simulink model "P2D_Overall"  (R2022a)
settings: Solver=VariableStepAuto  StartTime=0.0  StopTime=1  RelTol=1e-3
model workspace (MAT data in the model file):
  AN.EqPotentialHandle = 'E_eqGraphite'
  AN.i_oHandle = 'i_oC6'
  AN.sigmaHandle = 'sigmaC6'
  AN.D_oHandle = 'D_o_Graphite'
  AN.k_o = 3.80589129595e-09
  AN.alpha_a = 0.5
  AN.alpha_c = 0.5
  AN.C_dl = 3e-06
  AN.R_SEI = 0.00733702042142
  AN.sigma = 100
  AN.D_o = 3e-13
  AN.MW = 72.0642
  AN.MW_Lith = 79.0052
  AN.specCap = 350
  AN.rho = 2266
  AN.c_p = 720
  AN.k = 0.6
  AN.C_Li_max = 28.4851292094
  AN.del_z = 0.316227766017
  AN.del_y = 0.316227766017
  AN.L = 0.0001
  AN.r_p = 1.25e-05
  AN.eps_ed = 0.320700992698
  AN.eps_b = 0.172
  AN.A_geo = 1
  AN.gamma_brug = 1
  AN.alpha_brug = 1.5
  AN.del_x = 1e-05
  AN.x_vec = [5e-06 1.5e-05 2.5e-05 3.5e-05 4.5e-05 5.5e-05 6.5e-05 7.5e-05 8.5e-05 9.5e-05]
  AN.x_half_vec = [0 1e-05 2e-05 3e-05 4e-05 5e-05 6e-05 7e-05 8e-05 9e-05 0.0001]
  AN.del_r = 1.25e-06
  AN.r_vec = [6.25e-07 1.875e-06 3.125e-06 4.375e-06 5.625e-06 6.875e-06 8.125e-06 9.375e-06 1.0625e-05 1.1875e-05]
  AN.r_half_vec = [0 1.25e-06 2.5e-06 3.75e-06 5e-06 6.25e-06 7.5e-06 8.75e-06 1e-05 1.125e-05 1.25e-05]
  AN.eps_el = 0.507299007302
  AN.A_c = 0.1
  AN.Vol = 1e-05
  AN.dVol = 1e-06
  AN.V_sphere = 8.18123086872e-15
  AN.V_ed = 3.20700992698e-06
  AN.V_el = 5.07299007302e-06
  AN.dVol_el = 5.07299007302e-07
  AN.Np_tot = 391996018.501
  AN.Np_CV = 39199601.8501
  AN.A_surf = 1.96349540849e-09
  AN.A_surf_tot = 0.769682382475
  AN.A_surf_CV = 0.0769682382475
  AN.A_s = 76968.2382475
  AN.dVol_r = [8.18123086872e-18; 5.72686160811e-17; 1.55443386506e-16; 3.02705542143e-16; 4.99055082992e-16; 7.44492009054e-16; 1.03901632033e-15; 1.38262801681e-15; 1.77532709851e-15; 2.21711356542e-15]
  AN.Cap = 2.44837153197
  A_ROM = [0.499929926021  0.500277672565  -0.0239600367005  -0.00259805630083  0.0203144018753  -0.00104534668098  0.00239552572438  -0.000195556886825  -0.000910447986479  -7.26333553818e-05; -0.499881297031  -0.499911034591  -0.0239719306113  -0.00260057015341  0.0203228961157  -0.00104589940542  0.00239669880443  -0.000195607988547  -0.000910809830954  -7.2671508135e-05; 0.0251047076349  -0.0250959457318  0.987171638248  -0.00653392621931  0.0197762134396  -0.00226585752594  0.00331411596577  -0.000147058370919  -0.00053836838787  -4.66457939345e-05; -0.00955893642669  0.00955505732616  0.0123516491588  1.00099526202  -0.000703718615196  -0.000890966549299  0.00221912313357  -0.000101956509457  7.04769385898e-06  -4.36093200247e-06; 0.0212890549632  -0.0212815772566  -0.0230812878959  0.0308592552326  0.873793995824  -0.00311715755808  -0.0172138406461  0.00328787148246  0.0140204587776  0.001112904288; 0.00443110495424  -0.0044294863981  -0.0044884586816  0.00438260533447  -0.0577192270273  0.812800487273  0.104548665471  0.0343410474239  0.0440871519918  0.00415412252809; -0.00321407179364  0.00321296141751  0.00318368985247  -0.00520269619945  0.040746062799  0.244510956525  0.815824906709  -0.0403403883233  -0.00463968834278  0.000324235347067; 0.000411908248218  -0.000411728572718  -0.000450970628534  -0.000520935242046  -0.00616085036225  -0.0459578894952  0.0901889133124  0.991986422474  -0.0379589014963  -0.00193613802868; -0.000841734726446  0.000841438210464  0.000843091769749  -0.00117615267803  0.0106356056607  0.0898474768325  -0.118952953028  0.086084355624  0.424203198737  -0.0291971042377; -7.03725269776e-05  7.03386483629e-05  8.0548900339e-05  0.000189879859473  0.00113672762497  0.00528200920844  -0.0130569138272  -0.00245106078529  -0.137785624495  0.985398155877]
  A_est = [0.499929926021  0.500277672565  -0.0239600367005  -0.00259805630083  0.0203144018753  -0.00104534668098  0.00239552572438  -0.000195556886825  -0.000910447986479  -7.26333553818e-05; -0.499881297031  -0.499911034591  -0.0239719306113  -0.00260057015341  0.0203228961157  -0.00104589940542  0.00239669880443  -0.000195607988547  -0.000910809830954  -7.2671508135e-05; 0.0251047076349  -0.0250959457318  0.987171638248  -0.00653392621931  0.0197762134396  -0.00226585752594  0.00331411596577  -0.000147058370919  -0.00053836838787  -4.66457939345e-05; -0.00955893642669  0.00955505732616  0.0123516491588  1.00099526202  -0.000703718615196  -0.000890966549299  0.00221912313357  -0.000101956509457  7.04769385898e-06  -4.36093200247e-06; 0.0212890549632  -0.0212815772566  -0.0230812878959  0.0308592552326  0.873793995824  -0.00311715755808  -0.0172138406461  0.00328787148246  0.0140204587776  0.001112904288; 0.00443110495424  -0.0044294863981  -0.0044884586816  0.00438260533447  -0.0577192270273  0.812800487273  0.104548665471  0.0343410474239  0.0440871519918  0.00415412252809; -0.00321407179364  0.00321296141751  0.00318368985247  -0.00520269619945  0.040746062799  0.244510956525  0.815824906709  -0.0403403883233  -0.00463968834278  0.000324235347067; 0.000411908248218  -0.000411728572718  -0.000450970628534  -0.000520935242046  -0.00616085036225  -0.0459578894952  0.0901889133124  0.991986422474  -0.0379589014963  -0.00193613802868; -0.000841734726446  0.000841438210464  0.000843091769749  -0.00117615267803  0.0106356056607  0.0898474768325  -0.118952953028  0.086084355624  0.424203198737  -0.0291971042377; -7.03725269776e-05  7.03386483629e-05  8.0548900339e-05  0.000189879859473  0.00113672762497  0.00528200920844  -0.0130569138272  -0.00245106078529  -0.137785624495  0.985398155877]
  B_ROM = [0.250272154511; 0.25037068325; 0.000587633015339; 2.64174643029e-05; -4.66234471071e-05; 1.60139296354e-07; -1.87943663585e-07; -2.31065441941e-09; 7.21267341548e-09; 1.30921415116e-10]
  B_est = [0.250272154511; 0.25037068325; 0.000587633015339; 2.64174643029e-05; -4.66234471071e-05; 1.60139296354e-07; -1.87943663585e-07; -2.31065441941e-09; 7.21267341548e-09; 1.30921415116e-10]
  CA.EqPotentialHandle = 'E_eqNMC'
  CA.i_oHandle = 'i_oC6'
  CA.sigmaHandle = 'sigmaNMC'
  CA.D_oHandle = 'D_o_NMC532'
  CA.k_o = 9.72997022034e-10
  CA.alpha_a = 0.5
  CA.alpha_c = 0.5
  CA.C_dl = 1e-06
  CA.R_SEI = 0.00611911635272
  CA.sigma = 3.8
  CA.D_o = 5e-13
  CA.MW = 89.61275
  CA.MW_Lith = 96.55375
  CA.specCap = 170
  CA.rho = 2739.6961
  CA.c_p = 720
  CA.k = 0.6
  CA.C_Li_max = 40.5441490868
  CA.del_z = 0.316227766017
  CA.del_y = 0.316227766017
  CA.L = 0.0001
  CA.r_p = 5e-06
  CA.eps_ed = 0.442994582877
  CA.eps_b = 0.259
  CA.A_geo = 1
  CA.gamma_brug = 1
  CA.alpha_brug = 1.5
  CA.del_x = 1e-05
  CA.x_vec = [0.000135 0.000145 0.000155 0.000165 0.000175 0.000185 0.000195 0.000205 0.000215 0.000225]
  CA.x_half_vec = [0.00013 0.00014 0.00015 0.00016 0.00017 0.00018 0.00019 0.0002 0.00021 0.00022 0.00023]
  CA.del_r = 5e-07
  CA.r_vec = [2.5e-07 7.5e-07 1.25e-06 1.75e-06 2.25e-06 2.75e-06 3.25e-06 3.75e-06 4.25e-06 4.75e-06]
  CA.r_half_vec = [0 5e-07 1e-06 1.5e-06 2e-06 2.5e-06 3e-06 3.5e-06 4e-06 4.5e-06 5e-06]
  CA.eps_el = 0.298005417123
  CA.A_c = 0.1
  CA.Vol = 1e-05
  CA.dVol = 1e-06
  CA.V_sphere = 5.23598775598e-16
  CA.V_ed = 4.42994582877e-06
  CA.V_el = 2.98005417123e-06
  CA.dVol_el = 2.98005417123e-07
  CA.Np_tot = 8460573315.33
  CA.Np_CV = 846057331.533
  CA.A_surf = 3.14159265359e-10
  CA.A_surf_tot = 2.65796749726
  CA.A_surf_CV = 0.265796749726
  CA.A_s = 265796.749726
  CA.dVol_r = [5.23598775598e-19; 3.66519142919e-18; 9.94837673637e-18; 1.93731546971e-17; 3.19395253115e-17; 4.76474885794e-17; 6.6497044501e-17; 8.84881930761e-17; 1.13620934305e-16; 1.41895268187e-16]
  CA.Cap = 4.81377102891
  CONS.F = 96485338.3
  CONS.R = 8314.472
  CONS.T = 298.15
  C_ROM = [-0.00545632264226 0.00546070995292 -0.00275985407975 -0.0016343921732 -0.000623828440853 -0.00060095083733 0.000490320954801 1.36778683108e-05 0.000375099015739 1.69573705691e-05]
  C_est = [-0.00545632264226 0.00546070995292 -0.00275985407975 -0.0016343921732 -0.000623828440853 -0.00060095083733 0.000490320954801 1.36778683108e-05 0.000375099015739 1.69573705691e-05]
  C_plant = [0 0 -1 0 0 0 0 0 0 0 0 0 0 0 0 0 0 0 0 0 0 0 0 0 0 0 0 0 0 0 0 0 0 0 0 0 0 0 0 0 0 0 0 0 0 0 0 0 0 0 0 0 0 0 0 0 0 0 0 0 0 0 0 0 0 0 0 0 0 0 0 0 0 0 0 0 0 0 0 0 0 0 0 0 0 0 0 0 0 0 0 0 0 0 0 0 0 0 0 0 0 0 0 0 0 0 0 0 0 0 0 0 0 0 0 0 0 0 0 0 0 0 0 0 0 0 0 0 0 0 0 0 0 0 0 0 0 0 0 0 0 0 0 0 0 0 0 0 0 0 0 0 0 0 0 0 0 0 0 0 0 0 0 0 0 0 0 0 0 0 0 0 0 0 0 0 0 0 0 0 0 0 0 0 0 0 0 0 0 0 0 0 0 0 0 0 0 0 0 0 0 0 0 0 0 0 0 0 0 0 0 0 0 0 0 0 0 0 0 0 0 0 0 0 0 0 0 0 0 0 0 0 0 0 0 0 0 0 0 0 0 0 0 0 0 0 0 0 0 0 0 0 0 0 0 0 0 0 0 0 0 0 0 0 0 0 0 0 0 0 0 0 0 0 0 0 0 0 0 0 0 0 0 0 0 0 0 0 0 0 0 0 0 0 0 0 0 0 0 0 0 0 0 0 0 0 0 0 0 0 0 0 0 0 0 0 0 0 0 0 0 0 0 0 0 0 0 0 0 0 0 0 0 0 0 0 0 0 0 0 1 0 0 0 0 0 0 0 0 0 0 0 0 0 0]
  EL.tf_numHandle = 'transferenceNumber'
  EL.ActivityHandle = 'activity'
  EL.D_o_Li_ionHandle = 'D_oLiion'
  EL.kappaHandle = 'kappa'
  EL.D_o_Li_ion = 7.5e-11
  EL.kappa = 0.28
  EL.C = 1
  EL.tf_num = 0.363
  EL.Activity = 1
  EL.rho = 2266
  EL.c_p = 720
  EL.k = 470
  EL.gamma_brug = 1
  EL.alpha_brug = 1.5
  FLAG.AN_LI_FOIL = 0
  FLAG.CA_LI_FOIL = 0
  FLAG.R_AN = 1
  FLAG.R_CA = 1
  FLAG.COE = 0
  FLAG.T_BC_AN = 4
  FLAG.T_BC_CA = 4
  FLAG.CV_CONV = 0
  FLAG.HEAT_GEN_TOTAL = 1
  FLAG.HEAT_GEN_IONIC = 1
  FLAG.HEAT_GEN_ELECTRIC = 1
  FLAG.HEAT_GEN_RXN = 1
  FLAG.HEAT_GEN_CHEM_RXN = 0
  FLAG.V_SEI = 1
  FLAG.SEI_growth = 0
  FLAG.HeatGen = 0
  FLAG.Bruggeman = 0
  FLAG.BRUG_ED = 1
  FLAG.BRUG_EL = 1
  FLAG.BRUG_sigma = 1
  FLAG.BRUG_kappa = 1
  FLAG.BRUG_activity = 0
  FLAG.BRUG_D_Liion = 1
  FLAG.BRUG_tf_num = 0
  FLAG.BRUG_D_o_AN = 0
  FLAG.BRUG_D_o_CA = 0
  FLAG.Newman_i_o = 1
  FLAG.preDefined_C_max = 1
  FLAG.CONSTANT_PROPS_FROM_HANDLES = 0
  FLAG.VARIABLE_PROPS_FROM_HANDLES = 0
  FLAG.VARIABLE_kappa = 1
  FLAG.VARIABLE_activity = 0
  FLAG.VARIABLE_D_Liion = 0
  FLAG.VARIABLE_tf_num = 0
  FLAG.VARIABLE_D_o_AN = 0
  FLAG.VARIABLE_D_o_CA = 0
  FLAG.SaveSolnDiscreteTime = 1
  FLAG.SaveSystemForEst = 0
  FLAG.doPostProcessing = 1
  FLAG.ReduceSolnTime = 0
  FLAG.Plot = 0
  FLAG.PRBS_predefinded = 0
  Iden = [1  0  0  0  0  0  0  0  0  0; 0  1  0  0  0  0  0  0  0  0; 0  0  1  0  0  0  0  0  0  0; 0  0  0  1  0  0  0  0  0  0; 0  0  0  0  1  0  0  0  0  0; 0  0  0  0  0  1  0  0  0  0; 0  0  0  0  0  0  1  0  0  0; 0  0  0  0  0  0  0  1  0  0; 0  0  0  0  0  0  0  0  1  0; 0  0  0  0  0  0  0  0  0  1]
  K_infty = [-0.000684846249959; 0.000684373383459; -1.01289561233e-05; -0.00011865519077; -3.2008566389e-05; 3.30991855264e-05; 2.44710730896e-05; 6.82265210566e-05; 2.12049763989e-05; -0.000221635890042]
  K_plant = [0 0 0 0 0 0 0 0 0 0 0 0 ... (126025 elements, 355x355)]
  M_cross = [1 0 0 0 0 0 0 0 0 0 0 0 ... (126025 elements, 355x355)]
  N.N_CV_AN = 10
  N.N_CV_SEP = 5
  N.N_CV_CA = 10
  N.N_R_AN = 10
  N.N_R_CA = 10
  N.N_R_max = 10
  N.N_ES_var = 6
  N.N_SV_nR = 7
  N.N_SV_SEP = 3
  N.N_prop = 19
  N.N_SV_AN = 17
  N.N_SV_CA = 17
  N.N_SV_AN_tot = 170
  N.N_SV_SEP_tot = 15
  N.N_SV_CA_tot = 170
  N.N_SV_tot = 355
  N.N_CV_tot = 25
  N.CV_Region_AN = [1 2 3 4 5 6 7 8 9 10]
  N.CV_Region_SEP = [11 12 13 14 15]
  N.CV_Region_CA = [16 17 18 19 20 21 22 23 24 25]
  N.N_diff = 270
  N.N_algb = 85
  P.T = 1
  P.del_phi = 2
  P.phi_ed = 3
  P.V_1 = 4
  P.V_2 = 5
  P.i_PS = 6
  P.C_Liion = 7
  P.C_Li = 8
  P.C_Li_surf_AN = 17
  P.C_Li_surf_CA = 17
  P.C_Li_surf_max = 17
  P.SEP.T = 1
  P.SEP.phi_el = 2
  P.SEP.C_Liion = 3
  P.phi_el = 18
  P.ES.del_phi = 1
  P.ES.phi_ed = 2
  P.ES.V_1 = 3
  P.ES.V_2 = 4
  P.ES.i_PS = 5
  P.ES.i_dl = 6
  P.sigma = 1
  P.kappa = 2
  P.R_SEI = 3
  P.k = 4
  P.rho = 5
  P.c_p = 6
  P.D_o_Li_ion = 7
  P.activity = 8
  P.tf_num = 9
  P.D_o = 10
  PROPS = [100 0.28 0.00733702042142 0.6 2266 720 7.5e-11 1 0.363 3e-13 3e-13 3e-13 ... (475 elements, 19x25)]
  P_k_0 = [1  0  0  0  0  0  0  0  0  0; 0  1  0  0  0  0  0  0  0  0; 0  0  1  0  0  0  0  0  0  0; 0  0  0  1  0  0  0  0  0  0; 0  0  0  0  1  0  0  0  0  0; 0  0  0  0  0  1  0  0  0  0; 0  0  0  0  0  0  1  0  0  0; 0  0  0  0  0  0  0  1  0  0; 0  0  0  0  0  0  0  0  1  0; 0  0  0  0  0  0  0  0  0  1]
  Q = 1e-06
  R = 1e-06
  SEP.rho = 2266
  SEP.c_p = 720
  SEP.k = 0.6
  SEP.del_z = 0.316227766017
  SEP.del_y = 0.316227766017
  SEP.L = 3e-05
  SEP.eps = 1
  SEP.del_x = 6e-06
  SEP.x_vec = [0.000103 0.000109 0.000115 0.000121 0.000127]
  SEP.x_half_vec = [0.0001 0.000106 0.000112 0.000118 0.000124 0.00013]
  SEP.eps_el = 1
  SEP.A_c = 0.1
  SEP.Vol = 3e-06
  SEP.dVol = 6e-07
  SEP.V_el = 3e-06
  SEP.dVol_el = 6e-07
  SIM.results_filename = 'KalmanTest_KPCont_KalmanTestDTImpulseTs1.0SOC50.mat'
  SIM.SimMode = 4
  SIM.SOC_start = 50
  SIM.Ts = 1
  SIM.TsMultiple = 10
  SIM.SaveTimeStep = 0.1
  SIM.DiscreteTimeStep = 0.001
  SIM.ControllerHandle = 'Controller_CV'
  SIM.ZeroTime = 0.01
  SIM.cell_geo = 'p'
  SIM.Temp_start = 298.15
  SIM.T_inf = 298.15
  SIM.h = 1
  SIM.initial_offset = 0
  SIM.VoltageMax = 4.2
  SIM.VoltageMin = 3.4
  SIM.AnodeFormation_X = 0
  SIM.CathodeFormation_X = 1
  SIM.x_vec = [5e-06 1.5e-05 2.5e-05 3.5e-05 4.5e-05 5.5e-05 6.5e-05 7.5e-05 8.5e-05 9.5e-05 0.000103 0.000109 0.000115 0.000121 0.000127 0.000135 0.000145 0.000155 0.000165 0.000175 0.000185 0.000195 0.000205 0.000215 0.000225]
  SIM.x_half_vec = [0 1e-05 2e-05 3e-05 4e-05 5e-05 6e-05 7e-05 8e-05 9e-05 0.0001 0.000106 0.000112 0.000118 0.000124 0.00013 0.00014 0.00015 0.00016 0.00017 0.00018 0.00019 0.0002 0.00021 0.00022 0.00023]
  SIM.CV_vec = [1e-06 1e-06 1e-06 1e-06 1e-06 1e-06 1e-06 1e-06 1e-06 1e-06 6e-07 6e-07 6e-07 6e-07 6e-07 1e-06 1e-06 1e-06 1e-06 1e-06 1e-06 1e-06 1e-06 1e-06 1e-06]
  SIM.A_surf_CV_vec = [0.0769682382475 0.0769682382475 0.0769682382475 0.0769682382475 0.0769682382475 0.0769682382475 0.0769682382475 0.0769682382475 0.0769682382475 0.0769682382475 0 0 0 0 0 0.265796749726 0.265796749726 0.265796749726 0.265796749726 0.265796749726 0.265796749726 0.265796749726 0.265796749726 0.265796749726 0.265796749726]
  SIM.x_ini = 0.52035
  SIM.y_ini = 0.596540522221
  SIM.A_c = 0.1
  SIM.Cell_Cap = 2.44837153197
  SIM.current_MO_step = 3
  SIM.phi_guess = [0.10066050108; 0; -0.10066050108; -0.10066050108; 0; 0; 0.10066050108; 0; -0.10066050108; -0.10066050108; 0; 0; 0.10066050108; 0; -0.10066050108; -0.10066050108; 0; 0; 0.10066050108; 0; -0.10066050108; -0.10066050108; 0; 0; 0.10066050108; 0; -0.10066050108; -0.10066050108; 0; 0; 0.10066050108; 0; -0.10066050108; -0.10066050108; 0; 0; 0.10066050108; 0; -0.10066050108; -0.10066050108; 0; 0; 0.10066050108; 0; -0.10066050108; -0.10066050108; 0; 0; 0.10066050108; 0; -0.10066050108; -0.10066050108; 0; 0; 0.10066050108; 0; -0.10066050108; -0.10066050108; 0; 0; -0.10066050108; -0.10066050108; -0.10066050108; -0.10066050108; -0.10066050108; 3.84971530607; 3.74905480499; -0.10066050108; -0.10066050108; 0; 0; 3.84971530607; 3.74905480499; -0.10066050108; -0.10066050108; 0; 0; 3.84971530607; 3.74905480499; -0.10066050108; -0.10066050108; 0; 0; 3.84971530607; 3.74905480499; -0.10066050108; -0.10066050108; 0; 0; 3.84971530607; 3.74905480499; -0.10066050108; -0.10066050108; 0; 0; 3.84971530607; 3.74905480499; -0.10066050108; -0.10066050108; 0; 0; 3.84971530607; 3.74905480499; -0.10066050108; -0.10066050108; 0; 0; 3.84971530607; 3.74905480499; -0.10066050108; -0.10066050108; 0; 0; 3.84971530607; 3.74905480499; -0.10066050108; -0.10066050108; 0; 0; 3.84971530607; 3.74905480499; -0.10066050108; -0.10066050108; 0; 0; 0]
  SIM.SV_IC = [298.15 0.10066050108 0 -0.10066050108 -0.10066050108 0 1 14.8222369841 14.8222369841 14.8222369841 14.8222369841 14.8222369841 ... (355 elements, 355x1)]
  SIM.M = [1 0 0 0 0 0 0 0 0 0 0 0 ... (126025 elements, 355x355)]
  SIM.diff_idx = [1 2 7 8 9 10 11 12 13 14 15 16 17 18 19 24 25 26 27 28 29 30 31 32 33 34 35 36 41 42 43 44 45 46 47 48 49 50 51 52 53 58 59 60 61 62 63 64 65 66 67 68 69 70 75 76 77 78 79 80 81 82 83 84 85 86 87 92 93 94 95 96 97 98 99 100 101 102 103 104 109 110 111 112 113 114 115 116 117 118 119 120 121 126 127 128 129 130 131 132 133 134 135 136 137 138 143 144 145 146 147 148 149 150 151 152 153 154 155 160 161 162 163 164 165 166 167 168 169 170 171 173 174 176 177 179 180 182 183 185 186 187 192 193 194 195 196 197 198 199 200 201 202 203 204 209 210 211 212 213 214 215 216 217 218 219 220 221 226 227 228 229 230 231 232 233 234 235 236 237 238 243 244 245 246 247 248 249 250 251 252 253 254 255 260 261 262 263 264 265 266 267 268 269 270 271 272 277 278 279 280 281 282 283 284 285 286 287 288 289 294 295 296 297 298 299 300 301 302 303 304 305 306 311 312 313 314 315 316 317 318 319 320 321 322 323 328 329 330 331 332 333 334 335 336 337 338 339 340 345 346 347 348 349 350 351 352 353 354 355]
  SIM.algb_idx = [3 4 5 6 20 21 22 23 37 38 39 40 54 55 56 57 71 72 73 74 88 89 90 91 105 106 107 108 122 123 124 125 139 140 141 142 156 157 158 159 172 175 178 181 184 188 189 190 191 205 206 207 208 222 223 224 225 239 240 241 242 256 257 258 259 273 274 275 276 290 291 292 293 307 308 309 310 324 325 326 327 341 342 343 344]
  SIM.tSimEnd = 1.9786381
  SV_IC = [298.15 0.10066050108 0 -0.10066050108 -0.10066050108 0 1 14.8222369841 14.8222369841 14.8222369841 14.8222369841 14.8222369841 ... (355 elements, 355x1)]
  Ts = 1
  Ts_noise = 10
  U_NV_NT = [0 0 0 0 0 0 0 0 0 0 0 0 ... (126025 elements, 355x355)]
  pow_Q = 1e-05
  pow_R = 1e-05
  step_amp = 1
  step_time = 2
  x0_ROM = [0; 0; 0; 0; 0; 0; 0; 0; 0; 0]
  x0_est = [0; 0; 0; 0; 0; 0; 0; 0; 0; 0]
settings Model: Creator=tyevans  LastModifiedBy=tyevans

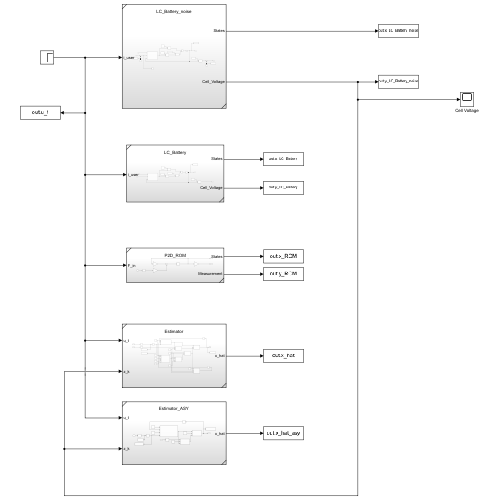
[thumbnail: Simulink's stored preview of the top-level diagram]
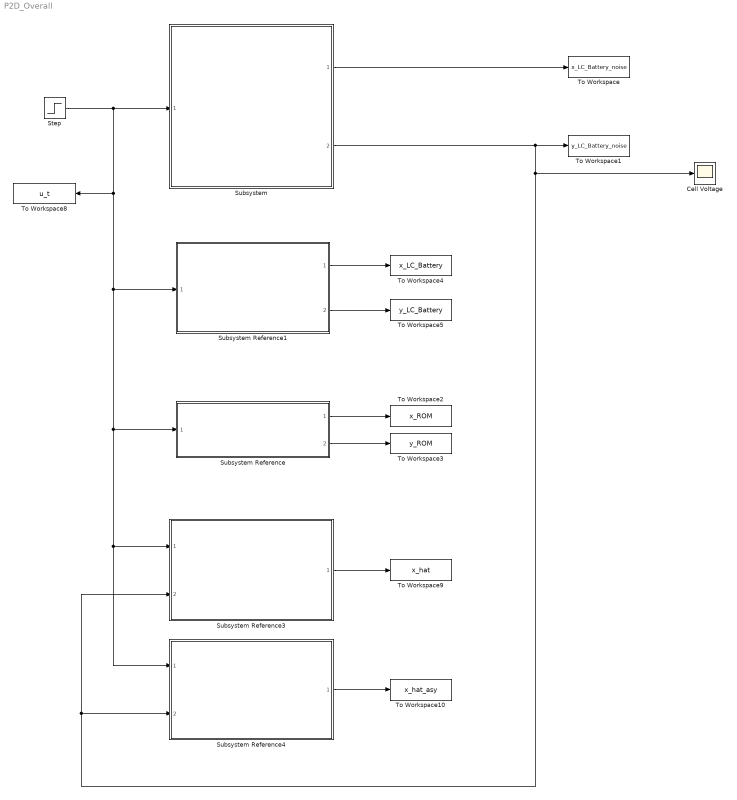
== system P2D_Overall ==
  Cell Voltage : Scope
  Step : Step  Time=step_time  After=step_amp  SampleTime=0
  Subsystem : Subsystem  ReferencedSubsystem=LC_Battery_noise
  Subsystem Reference : Subsystem  ReferencedSubsystem=P2D_ROM
  Subsystem Reference1 : Subsystem  ReferencedSubsystem=LC_Battery
  Subsystem Reference3 : Subsystem  ReferencedSubsystem=Estimator
  Subsystem Reference4 : Subsystem  ReferencedSubsystem=Estimator_ASY
  To Workspace : ToWorkspace  VariableName=x_LC_Battery_noise  SaveFormat=Structure With Time  SampleTime=-1
  To Workspace1 : ToWorkspace  VariableName=y_LC_Battery_noise  SaveFormat=Structure With Time  SampleTime=-1
  To Workspace10 : ToWorkspace  VariableName=x_hat_asy  SaveFormat=Structure With Time  SampleTime=-1
  To Workspace2 : ToWorkspace  VariableName=x_ROM  SaveFormat=Structure With Time  SampleTime=-1
  To Workspace3 : ToWorkspace  VariableName=y_ROM  SaveFormat=Structure With Time  SampleTime=-1
  To Workspace4 : ToWorkspace  VariableName=x_LC_Battery  SaveFormat=Structure With Time  SampleTime=-1
  To Workspace5 : ToWorkspace  VariableName=y_LC_Battery  SaveFormat=Structure With Time  SampleTime=-1
  To Workspace8 : ToWorkspace  VariableName=u_t  SaveFormat=Structure With Time  SampleTime=-1
  To Workspace9 : ToWorkspace  VariableName=x_hat  SaveFormat=Structure With Time  SampleTime=-1
  wires:
  Subsystem/1 -> To Workspace/1
  Subsystem/2 -> Cell Voltage/1, Subsystem Reference4/2, Subsystem Reference3/2, To Workspace1/1
  Subsystem Reference3/1 -> To Workspace9/1
  Step/1 -> To Workspace8/1, Subsystem Reference1/1, Subsystem Reference/1, Subsystem Reference4/1, Subsystem Reference3/1, Subsystem/1
  Subsystem Reference4/1 -> To Workspace10/1
  Subsystem Reference/1 -> To Workspace2/1
  Subsystem Reference/2 -> To Workspace3/1
  Subsystem Reference1/2 -> To Workspace5/1
  Subsystem Reference1/1 -> To Workspace4/1
